simulink model "ikincimodel"  (R2022b)
settings: Solver=VariableStepAuto  StartTime=0.0  StopTime=10.0  RelTol=1e-3
values from neighbouring files (symbols this model uses):
  K = 0.02    [Orantılı kontrol ile adım yanıtı.m]
  L = 0.5    [Orantılı kontrol ile adım yanıtı.m]
  R = 2    [Orantılı kontrol ile adım yanıtı.m]
settings Model: Creator=ardac  LastModifiedBy=ardac

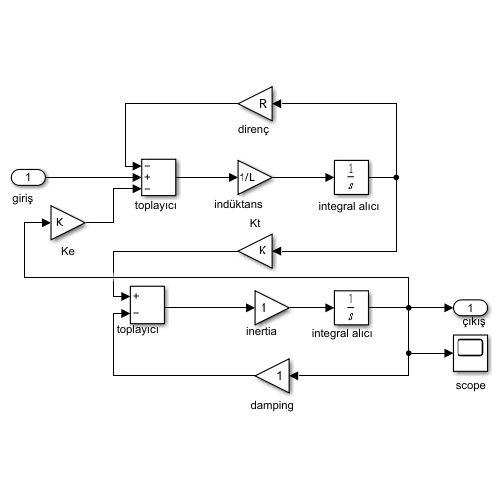
[thumbnail: Simulink's stored preview of the top-level diagram]
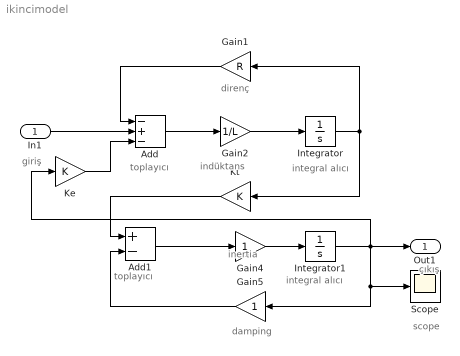
== system ikincimodel ==
  note: scope
  note: damping
  note: toplayıcı
  note: toplayıcı
  note: integral alıcı
  note: inertia
  note: çıkış
  note: giriş
  note: integral alıcı
  note: direnç
  note: indüktans
  In1 : Inport
  Add : Sum  Inputs=-+-
  Add1 : Sum  Inputs=+-
  Gain1 : Gain  Gain=R
  Gain2 : Gain  Gain=1/L
  Gain4 : Gain
  Gain5 : Gain
  Integrator : Integrator
  Integrator1 : Integrator
  Ke : Gain  Gain=K
  Kt : Gain  Gain=K
  Scope : Scope
  Out1 : Outport
  wires:
  In1/1 -> Add/2
  Gain1/1 -> Add/1
  Add/1 -> Gain2/1
  Ke/1 -> Add/3
  Gain2/1 -> Integrator/1
  Integrator/1 -> Gain1/1, Kt/1
  Kt/1 -> Add1/1
  Add1/1 -> Gain4/1
  Gain4/1 -> Integrator1/1
  Integrator1/1 -> Scope/1, Gain5/1, Ke/1, Out1/1
  Gain5/1 -> Add1/2
